simulink model "modestate32Calc"  (R2018b)
settings: Solver=FixedStepDiscrete  StartTime=0.0  StopTime=10.0  FixedStep=0.01  RelTol=1e-3
libraries: simulink x3
settings Model: Creator=sn2xws  LastModifiedBy=sn2xws
settings DataIOCC: SaveFormat=StructureWithTime
settings OptimizationCC: DefaultParameterBehavior=Inlined  EnhancedBackFolding=on  PassReuseOutputArgsAs=Individual arguments  ZeroExternalMemoryAtStartup=off  ZeroInternalMemoryAtStartup=off  OptimizeBlockOrder=speed  DifferentSizesBufferReuse=on  OptimizationCustomize=off
settings DebuggingCC: ParameterTunabilityLossMsg=error
settings ModelReferenceCC: ModelReferenceNumInstancesAllowed=Single
settings SFSimCC: MATLABDynamicMemAlloc=off
settings RTWCC: SystemTargetFile=autosar.tlc  GenCodeOnly=on  TemplateMakefile=ert_default_tmf  Description=AUTOSAR  GenerateReport=on  IncludeHyperlinkInReport=on  LaunchReport=on  GenerateTraceInfo=on  GenerateTraceReport=on  GenerateTraceReportSl=on  GenerateTraceReportSf=on  GenerateTraceReportEml=on  GenerateCodeMetricsReport=on
settings CodeAppCC: ForceParamTrailComments=on  IgnoreCustomStorageClasses=off  OperatorAnnotations=on  SimulinkDataObjDesc=on  SFDataObjDesc=on  InsertBlockDesc=on
settings STFCustomTargetCC: TargetLangStandard=C99 (ISO)  MultiwordLength=256  ParMdlRefBuildCompliant=on  CompOptLevelCompliant=on  IncludeMdlTerminateFcn=off  CombineOutputUpdateFcns=on  SuppressErrorStatus=on  ERTCustomFileBanners=on  SupportNonFinite=off  SupportComplex=off  SupportContinuousTime=off  SupportNonInlinedSFcns=off  RemoveResetFunc=on  MATLABClassNameForMDSCustomization=Simulink.SoftwareTarget.ERTCustomization  AutosarCompliant=on  UseToolchainInfoCompliant=on  LookupTableObjectStructAxisOrder=2,1,3,4,...  LUTObjectStructOrderEvenSpacing=Size,Table,Breakpoints  SystemTargetFile=autosar.tlc
settings ERTTargetCC: TargetLangStandard=C99 (ISO)  ConcurrentExecutionCompliant=off  IncludeMdlTerminateFcn=off  SuppressErrorStatus=on  SupportNonFinite=off  SupportComplex=off  ModelStepFunctionPrototypeControlCompliant=off  CPPClassGenCompliant=off  AutosarCompliant=on  LookupTableObjectStructAxisOrder=2,1,3,4,...  LUTObjectStructOrderEvenSpacing=Size,Table,Breakpoints  InlinedParameterPlacement=NonHierarchical  ERTCustomFileTemplate=example_file_process.tlc  ERTFilePackagingFormat=Compact

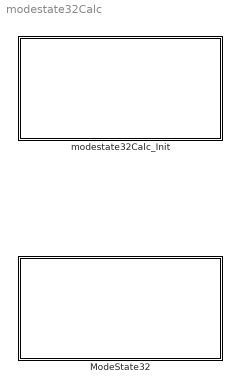
== system modestate32Calc ==
  ModeState32 : Subsystem
  modestate32Calc_Init : Subsystem

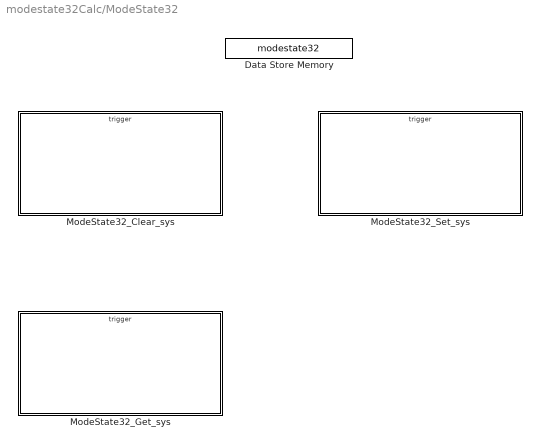
== system modestate32Calc/ModeState32 ==
  Data Store Memory : DataStoreMemory  DataStoreName=modestate32  ReadBeforeWriteMsg=warning  WriteAfterWriteMsg=warning  WriteAfterReadMsg=warning  ShowAdditionalParam=off
      settings: RTWStateStorageClass=ExportedGlobal
  ModeState32_Clear_sys : Subsystem
  ModeState32_Get_sys : Subsystem
  ModeState32_Set_sys : Subsystem

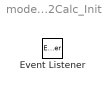
== system modestate32Calc/modestate32Calc_Init ==
  Event Listener : EventListener  EventName=reset

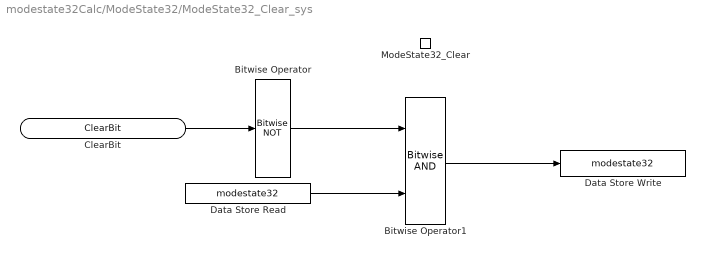
== system modestate32Calc/ModeState32/ModeState32_Clear_sys ==
  ModeState32_Clear : TriggerPort  TriggerType=function-call  IsSimulinkFunction=on  FunctionName=ModeState32_Clear  VariantControl=(inherit)
  Bitwise Operator : simulink/Logic and Bit Operations/Bitwise Operator  logicop=NOT  UseBitMask=off  BitMask=bin2dec('11011001')  BitMaskRealWorld=Stored Integer
  Bitwise Operator1 : simulink/Logic and Bit Operations/Bitwise Operator  logicop=AND  UseBitMask=off  NumInputPorts=2  BitMask=bin2dec('11011001')  BitMaskRealWorld=Stored Integer
  Data Store Read : DataStoreRead  DataStoreName=modestate32
  Data Store Write : DataStoreWrite  DataStoreName=modestate32
  ClearBit : ArgIn  OutDataTypeStr=uint32  ArgumentName=ClearBit
  wires:
  ClearBit/1 -> Bitwise Operator/1
  Bitwise Operator/1 -> Bitwise Operator1/1
  Data Store Read/1 -> Bitwise Operator1/2
  Bitwise Operator1/1 -> Data Store Write/1

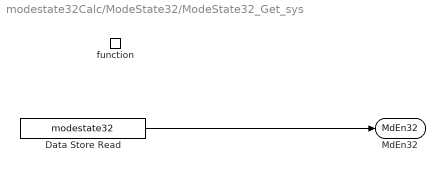
== system modestate32Calc/ModeState32/ModeState32_Get_sys ==
  function : TriggerPort  TriggerType=function-call  IsSimulinkFunction=on  FunctionName=ModeState32_Get  VariantControl=(inherit)
  Data Store Read : DataStoreRead  DataStoreName=modestate32
  MdEn32 : ArgOut  OutDataTypeStr=uint32  ArgumentName=MdEn32
  wires:
  Data Store Read/1 -> MdEn32/1

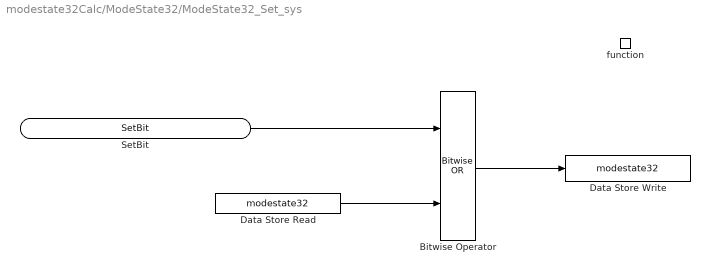
== system modestate32Calc/ModeState32/ModeState32_Set_sys ==
  function : TriggerPort  TriggerType=function-call  IsSimulinkFunction=on  FunctionName=ModeState32_Set  VariantControl=(inherit)
  Bitwise Operator : simulink/Logic and Bit Operations/Bitwise Operator  logicop=OR  UseBitMask=off  NumInputPorts=2  BitMask=bin2dec('11011001')  BitMaskRealWorld=Stored Integer
  Data Store Read : DataStoreRead  DataStoreName=modestate32
  Data Store Write : DataStoreWrite  DataStoreName=modestate32
  SetBit : ArgIn  OutDataTypeStr=uint32  ArgumentName=SetBit
  wires:
  SetBit/1 -> Bitwise Operator/1
  Data Store Read/1 -> Bitwise Operator/2
  Bitwise Operator/1 -> Data Store Write/1
